simulink model "IEEE9Buses"  (R2024b)
settings: Solver=FixedStepAuto  StartTime=0  StopTime=5  FixedStep=1e-6  RelTol=1e-3
values from neighbouring files (symbols this model uses):
  SG_D_1_D = 0.01056    [SG9_parameters.m]
  SG_D_1_EnableSaturation = 0    [SG9_parameters.m]
  SG_D_1_f0 = 60    [SG9_parameters.m]
  SG_D_1_H = 7.5    [SG9_parameters.m]
  SG_D_1_K_A = 20    [SG9_parameters.m]
  SG_D_1_K_E = 1.000000e+1    (= 10)    [SG9_parameters.m]
  SG_D_1_K_F = 2.363    [SG9_parameters.m]
  SG_D_1_K_s = 5    [SG9_parameters.m]
  SG_D_1_R_a = 0.001088    [SG9_parameters.m]
  SG_D_1_S_A = 1    [SG9_parameters.m]
  SG_D_1_S_B = 0.103    [SG9_parameters.m]
  SG_D_1_S_N = 10.659857    [SG9_parameters.m]
  SG_D_1_SpeedPara = 200    [SG9_parameters.m]
  SG_D_1_T_0 = 0.720173    [SG9_parameters.m]
  SG_D_1_T_1 = 0.3    [SG9_parameters.m]
  SG_D_1_T_2 = 0.05    [SG9_parameters.m]
  SG_D_1_T_3 = 0.02    [SG9_parameters.m]
  SG_D_1_T_4 = 0.005    [SG9_parameters.m]
  SG_D_1_T_A = 0.02    [SG9_parameters.m]
  SG_D_1_T_dd = 8.000000e+0    (= 8)    [SG9_parameters.m]
  SG_D_1_T_ddd = 0.04    [SG9_parameters.m]
  SG_D_1_T_E = 0.314    [SG9_parameters.m]
  SG_D_1_T_F = 0.35    [SG9_parameters.m]
  SG_D_1_T_qd = 0.8    [SG9_parameters.m]
  SG_D_1_T_qdd = 0.02    [SG9_parameters.m]
  SG_D_1_T_speed = 0.1    [SG9_parameters.m]
  SG_D_1_T_w = 0.5    [SG9_parameters.m]
  SG_D_1_V_ref = 1.990276    [SG9_parameters.m]
  SG_D_1_w_ref = 376.991118    [SG9_parameters.m]
  SG_D_1_x_d = 1.9    [SG9_parameters.m]
  SG_D_1_x_dd = 0.302    [SG9_parameters.m]
  SG_D_1_x_ddd = 0.204    [SG9_parameters.m]
  SG_D_1_x_l = 0.05    [SG9_parameters.m]
  SG_D_1_x_q = 1.3    [SG9_parameters.m]
  SG_D_1_x_qd = 0.5    [SG9_parameters.m]
  SG_D_1_x_qdd = 0.3    [SG9_parameters.m]
  SG_D_2_D = 0.01056    [SG9_parameters.m]
  SG_D_2_EnableSaturation = 0    [SG9_parameters.m]
  SG_D_2_f0 = 60    [SG9_parameters.m]
  SG_D_2_H = 7.5    [SG9_parameters.m]
  SG_D_2_K_A = 20    [SG9_parameters.m]
  SG_D_2_K_E = 1.000000e+1    (= 10)    [SG9_parameters.m]
  SG_D_2_K_F = 2.363    [SG9_parameters.m]
  SG_D_2_K_s = 0.5    [SG9_parameters.m]
  SG_D_2_R_a = 0.001088    [SG9_parameters.m]
  SG_D_2_S_A = 1    [SG9_parameters.m]
  SG_D_2_S_B = 0.103    [SG9_parameters.m]
  SG_D_2_S_N = 10.659857    [SG9_parameters.m]
  SG_D_2_SpeedPara = 200    [SG9_parameters.m]
  SG_D_2_T_0 = 1.632913    [SG9_parameters.m]
  SG_D_2_T_1 = 0.2    [SG9_parameters.m]
  SG_D_2_T_2 = 0.05    [SG9_parameters.m]
  SG_D_2_T_3 = 0.02    [SG9_parameters.m]
  SG_D_2_T_4 = 0.005    [SG9_parameters.m]
  SG_D_2_T_A = 0.02    [SG9_parameters.m]
  SG_D_2_T_dd = 8.000000e+0    (= 8)    [SG9_parameters.m]
  SG_D_2_T_ddd = 0.04    [SG9_parameters.m]
  SG_D_2_T_E = 0.314    [SG9_parameters.m]
  SG_D_2_T_F = 0.35    [SG9_parameters.m]
  SG_D_2_T_qd = 0.8    [SG9_parameters.m]
  SG_D_2_T_qdd = 0.02    [SG9_parameters.m]
  SG_D_2_T_speed = 0.1    [SG9_parameters.m]
  SG_D_2_T_w = 0.5    [SG9_parameters.m]
  SG_D_2_V_ref = 2.662631    [SG9_parameters.m]
  SG_D_2_w_ref = 376.991118    [SG9_parameters.m]
  SG_D_2_x_d = 1.9    [SG9_parameters.m]
  SG_D_2_x_dd = 0.302    [SG9_parameters.m]
  SG_D_2_x_ddd = 0.204    [SG9_parameters.m]
  SG_D_2_x_l = 0.05    [SG9_parameters.m]
  SG_D_2_x_q = 1.3    [SG9_parameters.m]
  SG_D_2_x_qd = 0.5    [SG9_parameters.m]
  SG_D_2_x_qdd = 0.3    [SG9_parameters.m]
  SG_D_3_D = 0.01056    [SG9_parameters.m]
  SG_D_3_EnableSaturation = 0    [SG9_parameters.m]
  SG_D_3_f0 = 60    [SG9_parameters.m]
  SG_D_3_H = 7.5    [SG9_parameters.m]
  SG_D_3_K_A = 20    [SG9_parameters.m]
  SG_D_3_K_E = 1.000000e+1    (= 10)    [SG9_parameters.m]
  SG_D_3_K_F = 2.363    [SG9_parameters.m]
  SG_D_3_K_s = 0.5    [SG9_parameters.m]
  SG_D_3_R_a = 0.001088    [SG9_parameters.m]
  SG_D_3_S_A = 1    [SG9_parameters.m]
  SG_D_3_S_B = 0.103    [SG9_parameters.m]
  SG_D_3_S_N = 10.659857    [SG9_parameters.m]
  SG_D_3_SpeedPara = 200    [SG9_parameters.m]
  SG_D_3_T_0 = 0.850788    [SG9_parameters.m]
  SG_D_3_T_1 = 0.2    [SG9_parameters.m]
  SG_D_3_T_2 = 0.05    [SG9_parameters.m]
  SG_D_3_T_3 = 0.02    [SG9_parameters.m]
  SG_D_3_T_4 = 0.005    [SG9_parameters.m]
  SG_D_3_T_A = 0.02    [SG9_parameters.m]
  SG_D_3_T_dd = 8.000000e+0    (= 8)    [SG9_parameters.m]
  SG_D_3_T_ddd = 0.04    [SG9_parameters.m]
  SG_D_3_T_E = 0.314    [SG9_parameters.m]
  SG_D_3_T_F = 0.35    [SG9_parameters.m]
  SG_D_3_T_qd = 0.8    [SG9_parameters.m]
  SG_D_3_T_qdd = 0.02    [SG9_parameters.m]
  SG_D_3_T_speed = 0.1    [SG9_parameters.m]
  SG_D_3_T_w = 0.5    [SG9_parameters.m]
  SG_D_3_V_ref = 1.915682    [SG9_parameters.m]
  SG_D_3_w_ref = 376.991118    [SG9_parameters.m]
  SG_D_3_x_d = 1.9    [SG9_parameters.m]
  SG_D_3_x_dd = 0.302    [SG9_parameters.m]
  SG_D_3_x_ddd = 0.204    [SG9_parameters.m]
  SG_D_3_x_l = 0.05    [SG9_parameters.m]
  SG_D_3_x_q = 1.3    [SG9_parameters.m]
  SG_D_3_x_qd = 0.5    [SG9_parameters.m]
  SG_D_3_x_qdd = 0.3    [SG9_parameters.m]
(part 4 of 9)

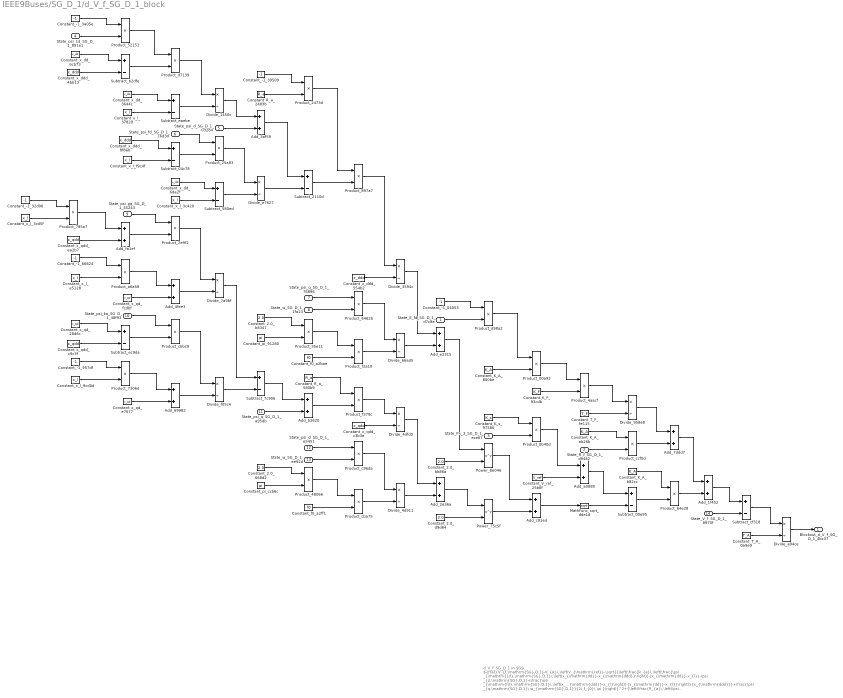
== system IEEE9Buses/SG_D_1/d_V_f_SG_D_1_block ==
  note: d_V_f_SG_D_1 in SG9
      | $-\frac{V_{f,\mathrm{SG},D,1}-K_{A}\,\left(V_{\mathrm{ref}}-\sqrt{{\left(\frac{R_{a}\,\left(\frac{\psi _{\mathrm{1d},\mathrm{SG},D,1}\,\left(x_{\mathrm{dd}}-x_{\mathrm{ddd}}\right)}{x_{\mathrm{dd}}-x_{l}}-\psi _{d,\mathrm{SG},D,1}+\frac{\psi _{\mathrm{fd},\mathrm{SG},D,1}\,\left(x_{\mathrm{ddd}}-x_{l}\right)}{x_{\mathrm{dd}}-x_{l}}\right)}{x_{\mathrm{ddd}}}+\frac{\psi _{q,\mathrm{SG},D,1}\,w_{\mathrm{SG},D,1}}{2\,f_{0}\,\pi }\right)}^2+{\left(\frac{R_{a}\,\left(\psi _{q,\mathrm{SG},D,1}+\frac{\psi _{\mathrm{gq},\mathrm{SG},D,1}\,\left(x_{l}-x_{\mathrm{qdd}}\right)}{x_{l}-x_{\mathrm{qd}}}+\frac{\psi _{\mathrm{kq},\mathrm{SG},D,1}\,\left(x_{\mathrm{qd}}-x_{\mathrm{qdd}}\right)}{x_{l}-x_{\mathrm{qd}}}\right)}{x_{\mathrm{qdd}}}+\frac{\psi _{d,\mathrm{SG},D,1}\,w_{\mathrm{SG},D,1}}{2\,f_{0}\,\pi }\right)}^2}+K_{s}\,\mathrm{Px}_{3,\mathrm{SG},D,1}\right)-K_{A}\,R_{f,\mathrm{SG},D,1}+\frac{E_{\mathrm{fd},\mathrm{SG},D,1}\,K_{A}\,K_{F}}{T_{F}}}{T_{A}}$
      | Automatically generated on 2025-09-12 21:31:27 .
  State_E_fd_SG_D_1_d7c8e : Inport
  State_R_f_SG_D_1_d9482 : Inport  Port=2
  State_Px_3_SG_D_1_ece67 : Inport  Port=3
  State_psi_1d_SG_D_1_891e1 : Inport  Port=4
  State_psi_d_SG_D_1_03284 : Inport  Port=5
  State_psi_fd_SG_D_1_16d3d : Inport  Port=6
  State_psi_q_SG_D_1_76896 : Inport  Port=7
  State_w_SG_D_1_1fa23 : Inport  Port=8
  State_psi_gq_SG_D_1_45243 : Inport  Port=9
  State_psi_kq_SG_D_1_48f93 : Inport  Port=10
  State_psi_q_SG_D_1_a95db : Inport  Port=11
  State_psi_d_SG_D_1_e5451 : Inport  Port=12
  State_w_SG_D_1_ee92d : Inport  Port=13
  State_V_f_SG_D_1_8970f : Inport  Port=14
  Add_1f452 : Sum
  Add_2e36a : Sum
  Add_3af59 : Sum
  Add_4fee3 : Sum
  Add_69982 : Sum
  Add_7ddd7 : Sum
  Add_a0880 : Sum
  Add_b2620 : Sum
  Add_c91ed : Sum
  Add_e2315 : Sum
  Add_fa1ef : Sum
  Constant_-1_04053 : Constant  Value=-1
  Constant_-1_32d06 : Constant  Value=-1
  Constant_-1_39509 : Constant  Value=-1
  Constant_-1_3a05e : Constant  Value=-1
  Constant_-1_66824 : Constant  Value=-1
  Constant_-1_957df : Constant  Value=-1
  Constant_2.0_668d2 : Constant  Value=2.0
  Constant_2.0_b8347 : Constant  Value=2.0
  Constant_2.0_bb86a : Constant  Value=2.0
  Constant_2.0_d9d64 : Constant  Value=2.0
  Constant_K_A_800be : Constant  Value=K_A
  Constant_K_A_ab26b : Constant  Value=K_A
  Constant_K_A_b82cc : Constant  Value=K_A
  Constant_K_F_93cdb : Constant  Value=K_F
  Constant_K_s_97580 : Constant  Value=K_s
  Constant_R_a_2483b : Constant  Value=R_a
  Constant_R_a_580b9 : Constant  Value=R_a
  Constant_T_A_0a9e9 : Constant  Value=T_A
  Constant_T_F_fe115 : Constant  Value=T_F
  Constant_V_ref_25b6f : Constant  Value=V_ref
  Constant_f0_a2bae : Constant  Value=f0
  Constant_f0_a2ff1 : Constant  Value=f0
  Constant_pi_91280 : Constant  Value=pi
  Constant_pi_ccb6c : Constant  Value=pi
  Constant_x_dd_3644c : Constant  Value=x_dd
  Constant_x_dd_6cb73 : Constant  Value=x_dd
  Constant_x_dd_6da2f : Constant  Value=x_dd
  Constant_x_ddd_4bb13 : Constant  Value=x_ddd
  Constant_x_ddd_554b2 : Constant  Value=x_ddd
  Constant_x_ddd_8f8ab : Constant  Value=x_ddd
  Constant_x_l_3782d : Constant  Value=x_l
  Constant_x_l_3c420 : Constant  Value=x_l
  Constant_x_l_3cd5f : Constant  Value=x_l
  Constant_x_l_9cd0d : Constant  Value=x_l
  Constant_x_l_e5128 : Constant  Value=x_l
  Constant_x_l_f9c4f : Constant  Value=x_l
  Constant_x_qd_28d6c : Constant  Value=x_qd
  Constant_x_qd_e7677 : Constant  Value=x_qd
  Constant_x_qd_fcdbf : Constant  Value=x_qd
  Constant_x_qdd_c3b3e : Constant  Value=x_qdd
  Constant_x_qdd_c9c3f : Constant  Value=x_qdd
  Constant_x_qdd_ea2b7 : Constant  Value=x_qdd
  Divide_1450c : Product  Inputs=*/
  Divide_3594c : Product  Inputs=*/
  Divide_4d911 : Product  Inputs=*/
  Divide_4dfd0 : Product  Inputs=*/
  Divide_66ad5 : Product  Inputs=*/
  Divide_7a9bf : Product  Inputs=*/
  Divide_958e8 : Product  Inputs=*/
  Divide_a94ce : Product  Inputs=*/
  Divide_e7627 : Product  Inputs=*/
  Divide_f05c4 : Product  Inputs=*/
  MathFunc_sqrt_dde1d : Sqrt
  Power_75c5f : Math  Operator=pow
  Power_8e046 : Math  Operator=pow
  Product_00a92 : Product
  Product_0b40d : Product
  Product_2473d : Product
  Product_25a83 : Product
  Product_2e9f2 : Product
  Product_35e11 : Product
  Product_48066 : Product
  Product_4aacf : Product
  Product_52151 : Product
  Product_6462b : Product
  Product_64e28 : Product
  Product_7306d : Product
  Product_785a7 : Product
  Product_897a7 : Product
  Product_a6a58 : Product
  Product_c96da : Product
  Product_cba75 : Product
  Product_cbbc9 : Product
  Product_ccf0d : Product
  Product_d7139 : Product
  Product_d98a2 : Product
  Product_f2a10 : Product
  Product_f379c : Product
  Subtract_00e95 : Sum  Inputs=+-
  Subtract_04c78 : Sum  Inputs=+-
  Subtract_2110d : Sum  Inputs=+-
  Subtract_580ed : Sum  Inputs=+-
  Subtract_7c906 : Sum  Inputs=+-
  Subtract_b2dfe : Sum  Inputs=+-
  Subtract_cf318 : Sum  Inputs=+-
  Subtract_eaebe : Sum  Inputs=+-
  Subtract_ec9da : Sum  Inputs=+-
  Blockout_d_V_f_SG_D_1_4bc37 : Outport
  wires:
  Constant_-1_957df/1 -> Product_7306d/1
  Constant_-1_32d06/1 -> Product_785a7/1
  State_psi_d_SG_D_1_e5451/1 -> Product_c96da/1
  Constant_x_qd_e7677/1 -> Add_69982/2
  Constant_x_qdd_ea2b7/1 -> Add_fa1ef/2
  State_w_SG_D_1_ee92d/1 -> Product_c96da/2
  Constant_x_l_3cd5f/1 -> Product_785a7/2
  Subtract_2110d/1 -> Product_897a7/2
  Constant_x_l_9cd0d/1 -> Product_7306d/2
  Constant_x_dd_6cb73/1 -> Subtract_b2dfe/1
  Constant_R_a_2483b/1 -> Product_2473d/2
  Constant_-1_3a05e/1 -> Product_52151/1
  Divide_e7627/1 -> Subtract_2110d/2
  Constant_x_ddd_4bb13/1 -> Subtract_b2dfe/2
  Add_69982/1 -> Divide_f05c4/2
  State_psi_1d_SG_D_1_891e1/1 -> Product_52151/2
  Add_4fee3/1 -> Divide_7a9bf/2
  Subtract_ec9da/1 -> Product_cbbc9/2
  Product_4aacf/1 -> Divide_958e8/1
  Product_35e11/1 -> Product_f2a10/1
  Product_785a7/1 -> Add_fa1ef/1
  Constant_-1_66824/1 -> Product_a6a58/1
  Constant_x_l_e5128/1 -> Product_a6a58/2
  Add_3af59/1 -> Subtract_2110d/1
  Constant_2.0_668d2/1 -> Product_48066/1
  Constant_x_qd_28d6c/1 -> Subtract_ec9da/1
  Product_52151/1 -> Product_d7139/1
  Constant_pi_ccb6c/1 -> Product_48066/2
  Constant_x_qdd_c9c3f/1 -> Subtract_ec9da/2
  Subtract_b2dfe/1 -> Product_d7139/2
  State_psi_q_SG_D_1_a95db/1 -> Add_b2620/2
  Constant_x_dd_3644c/1 -> Subtract_eaebe/1
  Constant_x_l_3782d/1 -> Subtract_eaebe/2
  Constant_x_ddd_8f8ab/1 -> Subtract_04c78/1
  Constant_x_l_f9c4f/1 -> Subtract_04c78/2
  State_psi_gq_SG_D_1_45243/1 -> Product_2e9f2/1
  Add_fa1ef/1 -> Product_2e9f2/2
  Product_a6a58/1 -> Add_4fee3/1
  Constant_x_qd_fcdbf/1 -> Add_4fee3/2
  Divide_1450c/1 -> Add_3af59/1
  Subtract_eaebe/1 -> Divide_1450c/2
  State_psi_kq_SG_D_1_48f93/1 -> Product_cbbc9/1
  Divide_a94ce/1 -> Blockout_d_V_f_SG_D_1_4bc37/1
  Product_7306d/1 -> Add_69982/1
  Product_d7139/1 -> Divide_1450c/1
  State_psi_fd_SG_D_1_16d3d/1 -> Product_25a83/1
  State_w_SG_D_1_1fa23/1 -> Product_6462b/2
  Subtract_04c78/1 -> Product_25a83/2
  Constant_x_dd_6da2f/1 -> Subtract_580ed/1
  Constant_x_l_3c420/1 -> Subtract_580ed/2
  Product_2e9f2/1 -> Divide_7a9bf/1
  Product_2473d/1 -> Product_897a7/1
  Product_cbbc9/1 -> Divide_f05c4/1
  State_psi_d_SG_D_1_03284/1 -> Add_3af59/2
  Product_25a83/1 -> Divide_e7627/1
  Subtract_580ed/1 -> Divide_e7627/2
  Divide_7a9bf/1 -> Subtract_7c906/1
  Divide_f05c4/1 -> Subtract_7c906/2
  Constant_-1_39509/1 -> Product_2473d/1
  Constant_2.0_b8347/1 -> Product_35e11/1
  Constant_pi_91280/1 -> Product_35e11/2
  Subtract_7c906/1 -> Add_b2620/1
  State_psi_q_SG_D_1_76896/1 -> Product_6462b/1
  Constant_f0_a2bae/1 -> Product_f2a10/2
  Constant_R_a_580b9/1 -> Product_f379c/1
  Add_b2620/1 -> Product_f379c/2
  Product_48066/1 -> Product_cba75/1
  Power_8e046/1 -> Add_c91ed/1
  Constant_f0_a2ff1/1 -> Product_cba75/2
  Product_897a7/1 -> Divide_3594c/1
  Constant_x_ddd_554b2/1 -> Divide_3594c/2
  Product_6462b/1 -> Divide_66ad5/1
  Product_f2a10/1 -> Divide_66ad5/2
  Product_f379c/1 -> Divide_4dfd0/1
  Constant_x_qdd_c3b3e/1 -> Divide_4dfd0/2
  Product_c96da/1 -> Divide_4d911/1
  Product_cba75/1 -> Divide_4d911/2
  Divide_3594c/1 -> Add_e2315/1
  Divide_66ad5/1 -> Add_e2315/2
  Divide_4dfd0/1 -> Add_2e36a/1
  Divide_4d911/1 -> Add_2e36a/2
  Constant_-1_04053/1 -> Product_d98a2/1
  State_E_fd_SG_D_1_d7c8e/1 -> Product_d98a2/2
  Add_e2315/1 -> Power_8e046/1
  Constant_2.0_bb86a/1 -> Power_8e046/2
  Add_2e36a/1 -> Power_75c5f/1
  Constant_2.0_d9d64/1 -> Power_75c5f/2
  Product_d98a2/1 -> Product_00a92/1
  Constant_K_A_800be/1 -> Product_00a92/2
  Constant_K_s_97580/1 -> Product_0b40d/1
  State_Px_3_SG_D_1_ece67/1 -> Product_0b40d/2
  Power_75c5f/1 -> Add_c91ed/2
  Divide_958e8/1 -> Add_7ddd7/1
  Product_00a92/1 -> Product_4aacf/1
  Constant_K_F_93cdb/1 -> Product_4aacf/2
  Product_0b40d/1 -> Add_a0880/1
  Constant_V_ref_25b6f/1 -> Add_a0880/2
  Add_c91ed/1 -> MathFunc_sqrt_dde1d/1
  Constant_T_F_fe115/1 -> Divide_958e8/2
  Constant_K_A_ab26b/1 -> Product_ccf0d/1
  State_R_f_SG_D_1_d9482/1 -> Product_ccf0d/2
  Add_a0880/1 -> Subtract_00e95/1
  MathFunc_sqrt_dde1d/1 -> Subtract_00e95/2
  Constant_T_A_0a9e9/1 -> Divide_a94ce/2
  Product_ccf0d/1 -> Add_7ddd7/2
  Constant_K_A_b82cc/1 -> Product_64e28/1
  Subtract_00e95/1 -> Product_64e28/2
  Add_7ddd7/1 -> Add_1f452/1
  Product_64e28/1 -> Add_1f452/2
  Add_1f452/1 -> Subtract_cf318/1
  State_V_f_SG_D_1_8970f/1 -> Subtract_cf318/2
  Subtract_cf318/1 -> Divide_a94ce/1

== system IEEE9Buses/SG_D_1/d_psi_1d_SG_D_1_block ==
  note: d_psi_1d_SG_D_1 in SG9
      | $-\frac{\psi _{\mathrm{1d},\mathrm{SG},D,1}-\psi _{\mathrm{fd},\mathrm{SG},D,1}+\frac{\left(x_{\mathrm{dd}}-x_{l}\right)\,\left(\frac{\psi _{\mathrm{1d},\mathrm{SG},D,1}\,\left(x_{\mathrm{dd}}-x_{\mathrm{ddd}}\right)}{x_{\mathrm{dd}}-x_{l}}-\psi _{d,\mathrm{SG},D,1}+\frac{\psi _{\mathrm{fd},\mathrm{SG},D,1}\,\left(x_{\mathrm{ddd}}-x_{l}\right)}{x_{\mathrm{dd}}-x_{l}}\right)}{x_{\mathrm{ddd}}}}{T_{\mathrm{ddd}}}$
      | Automatically generated on 2025-09-12 21:31:05 .
  State_psi_1d_SG_D_1_d2762 : Inport
  State_psi_fd_SG_D_1_bca21 : Inport  Port=2
  State_psi_1d_SG_D_1_c520a : Inport  Port=3
  State_psi_d_SG_D_1_3f3ac : Inport  Port=4
  State_psi_fd_SG_D_1_eccee : Inport  Port=5
  Add_b1279 : Sum
  Add_c201e : Sum
  Add_cfc23 : Sum
  Constant_-1_296e1 : Constant  Value=-1
  Constant_-1_5c271 : Constant  Value=-1
  Constant_T_ddd_caaec : Constant  Value=T_ddd
  Constant_x_dd_2b56b : Constant  Value=x_dd
  Constant_x_dd_87b87 : Constant  Value=x_dd
  Constant_x_dd_8f6dc : Constant  Value=x_dd
  Constant_x_dd_c90dd : Constant  Value=x_dd
  Constant_x_ddd_16ccc : Constant  Value=x_ddd
  Constant_x_ddd_bf0c4 : Constant  Value=x_ddd
  Constant_x_ddd_d1635 : Constant  Value=x_ddd
  Constant_x_l_09e53 : Constant  Value=x_l
  Constant_x_l_48004 : Constant  Value=x_l
  Constant_x_l_58458 : Constant  Value=x_l
  Constant_x_l_bfbd3 : Constant  Value=x_l
  Divide_2506c : Product  Inputs=*/
  Divide_70d34 : Product  Inputs=*/
  Divide_77283 : Product  Inputs=*/
  Divide_cc347 : Product  Inputs=*/
  Product_15131 : Product
  Product_1d398 : Product
  Product_2cf84 : Product
  Product_4a14f : Product
  Product_e7278 : Product
  Subtract_15a9f : Sum  Inputs=+-
  Subtract_1ef53 : Sum  Inputs=+-
  Subtract_30208 : Sum  Inputs=+-
  Subtract_aaa5c : Sum  Inputs=+-
  Subtract_b8043 : Sum  Inputs=+-
  Subtract_efad1 : Sum  Inputs=+-
  Blockout_d_psi_1d_SG_D_1_4de60 : Outport
  wires:
  Product_15131/1 -> Product_4a14f/1
  Constant_-1_296e1/1 -> Product_15131/1
  Subtract_1ef53/1 -> Product_4a14f/2
  State_psi_1d_SG_D_1_c520a/1 -> Product_15131/2
  Subtract_b8043/1 -> Product_e7278/1
  State_psi_d_SG_D_1_3f3ac/1 -> Add_b1279/2
  Constant_x_dd_2b56b/1 -> Subtract_15a9f/1
  Constant_x_l_09e53/1 -> Subtract_b8043/2
  Constant_x_dd_8f6dc/1 -> Subtract_1ef53/1
  Subtract_30208/1 -> Product_2cf84/2
  Constant_x_l_48004/1 -> Subtract_15a9f/2
  Divide_2506c/1 -> Subtract_efad1/2
  Constant_x_ddd_16ccc/1 -> Subtract_1ef53/2
  Constant_x_ddd_bf0c4/1 -> Subtract_30208/1
  Constant_x_l_bfbd3/1 -> Subtract_30208/2
  Add_cfc23/1 -> Add_c201e/1
  Product_4a14f/1 -> Divide_77283/1
  Divide_cc347/1 -> Add_c201e/2
  Subtract_15a9f/1 -> Divide_77283/2
  State_psi_fd_SG_D_1_eccee/1 -> Product_2cf84/1
  Constant_x_dd_c90dd/1 -> Subtract_aaa5c/1
  Constant_x_l_58458/1 -> Subtract_aaa5c/2
  Constant_x_ddd_d1635/1 -> Divide_cc347/2
  Subtract_efad1/1 -> Product_e7278/2
  Divide_77283/1 -> Add_b1279/1
  Product_2cf84/1 -> Divide_2506c/1
  Subtract_aaa5c/1 -> Divide_2506c/2
  Product_e7278/1 -> Divide_cc347/1
  Constant_x_dd_87b87/1 -> Subtract_b8043/1
  Add_b1279/1 -> Subtract_efad1/1
  Constant_-1_5c271/1 -> Product_1d398/1
  State_psi_1d_SG_D_1_d2762/1 -> Product_1d398/2
  Product_1d398/1 -> Add_cfc23/1
  State_psi_fd_SG_D_1_bca21/1 -> Add_cfc23/2
  Add_c201e/1 -> Divide_70d34/1
  Constant_T_ddd_caaec/1 -> Divide_70d34/2
  Divide_70d34/1 -> Blockout_d_psi_1d_SG_D_1_4de60/1

== system IEEE9Buses/SG_D_1/d_psi_d_SG_D_1_block ==
  note: d_psi_d_SG_D_1 in SG9
      | $2\,\pi \,f_{0}\,\left(v_{d,\mathrm{SG},D,1}\,\sin\left(\theta _{\mathrm{SG},D,1}\right)-v_{q,\mathrm{SG},D,1}\,\cos\left(\theta _{\mathrm{SG},D,1}\right)+\frac{R_{a}\,\left(\frac{\psi _{\mathrm{1d},\mathrm{SG},D,1}\,\left(x_{\mathrm{dd}}-x_{\mathrm{ddd}}\right)}{x_{\mathrm{dd}}-x_{l}}-\psi _{d,\mathrm{SG},D,1}+\frac{\psi _{\mathrm{fd},\mathrm{SG},D,1}\,\left(x_{\mathrm{ddd}}-x_{l}\right)}{x_{\mathrm{dd}}-x_{l}}\right)}{x_{\mathrm{ddd}}}+\frac{\psi _{q,\mathrm{SG},D,1}\,w_{\mathrm{SG},D,1}}{2\,f_{0}\,\pi }\right)$
      | Automatically generated on 2025-09-12 21:30:56 .
  State_psi_1d_SG_D_1_86041 : Inport
  State_psi_d_SG_D_1_dbe44 : Inport  Port=2
  State_psi_fd_SG_D_1_6e896 : Inport  Port=3
  Input_v_d_SG_D_1_19f90 : Inport  Port=4
  State_theta_SG_D_1_15a2a : Inport  Port=5
  Input_v_q_SG_D_1_67e4a : Inport  Port=6
  State_theta_SG_D_1_2debe : Inport  Port=7
  State_psi_q_SG_D_1_4f741 : Inport  Port=8
  State_w_SG_D_1_13bdb : Inport  Port=9
  Add_51bf5 : Sum
  Add_5a4e2 : Sum
  Constant_-1_86b72 : Constant  Value=-1
  Constant_-2.0_180c6 : Constant  Value=-2.0
  Constant_2.0_e7900 : Constant  Value=2.0
  Constant_R_a_4c0ac : Constant  Value=R_a
  Constant_f0_3c565 : Constant  Value=f0
  Constant_f0_a234f : Constant  Value=f0
  Constant_pi_33d76 : Constant  Value=pi
  Constant_pi_5f677 : Constant  Value=pi
  Constant_x_dd_5ee26 : Constant  Value=x_dd
  Constant_x_dd_bfc30 : Constant  Value=x_dd
  Constant_x_dd_dc9dd : Constant  Value=x_dd
  Constant_x_ddd_43fba : Constant  Value=x_ddd
  Constant_x_ddd_75169 : Constant  Value=x_ddd
  Constant_x_ddd_d754c : Constant  Value=x_ddd
  Constant_x_l_4ff12 : Constant  Value=x_l
  Constant_x_l_79896 : Constant  Value=x_l
  Constant_x_l_82ac6 : Constant  Value=x_l
  Divide_5216b : Product  Inputs=*/
  Divide_5b670 : Product  Inputs=*/
  Divide_816d9 : Product  Inputs=*/
  Divide_f246b : Product  Inputs=*/
  MathFunc_cos_15b49 : Trigonometry  Operator=cos
  MathFunc_sin_0787e : Trigonometry
  Product_06b68 : Product
  Product_11279 : Product
  Product_27c5b : Product
  Product_28ed5 : Product
  Product_3b359 : Product
  Product_3ce3c : Product
  Product_44fc3 : Product
  Product_70878 : Product
  Product_7e125 : Product
  Product_d0240 : Product
  Product_d34c7 : Product
  Product_f3a48 : Product
  Subtract_0408f : Sum  Inputs=+-
  Subtract_0ef44 : Sum  Inputs=+-
  Subtract_112a7 : Sum  Inputs=+-
  Subtract_4ad5b : Sum  Inputs=+-
  Subtract_54635 : Sum  Inputs=+-
  Subtract_78ef5 : Sum  Inputs=+-
  Subtract_c5ec9 : Sum  Inputs=+-
  Blockout_d_psi_d_SG_D_1_534f2 : Outport
  wires:
  Add_51bf5/1 -> Subtract_0ef44/1
  Product_d34c7/1 -> Divide_5b670/1
  Subtract_c5ec9/1 -> Product_d34c7/2
  Divide_5b670/1 -> Add_51bf5/1
  Product_27c5b/1 -> Product_d34c7/1
  Constant_x_ddd_d754c/1 -> Subtract_c5ec9/2
  Constant_x_dd_dc9dd/1 -> Subtract_c5ec9/1
  State_psi_1d_SG_D_1_86041/1 -> Product_27c5b/2
  Constant_-1_86b72/1 -> Product_27c5b/1
  Product_f3a48/1 -> Divide_f246b/1
  Constant_x_l_4ff12/1 -> Subtract_4ad5b/2
  State_psi_d_SG_D_1_dbe44/1 -> Add_51bf5/2
  Constant_x_dd_bfc30/1 -> Subtract_4ad5b/1
  Constant_x_ddd_43fba/1 -> Subtract_78ef5/1
  Constant_x_l_82ac6/1 -> Subtract_78ef5/2
  Subtract_4ad5b/1 -> Divide_5b670/2
  State_psi_fd_SG_D_1_6e896/1 -> Product_f3a48/1
  Constant_x_ddd_75169/1 -> Divide_816d9/2
  Subtract_78ef5/1 -> Product_f3a48/2
  Product_7e125/1 -> Subtract_112a7/2
  Constant_x_dd_5ee26/1 -> Subtract_54635/1
  Constant_x_l_79896/1 -> Subtract_54635/2
  Subtract_54635/1 -> Divide_f246b/2
  Divide_f246b/1 -> Subtract_0ef44/2
  Constant_R_a_4c0ac/1 -> Product_d0240/1
  Subtract_0ef44/1 -> Product_d0240/2
  MathFunc_cos_15b49/1 -> Product_44fc3/2
  State_theta_SG_D_1_15a2a/1 -> MathFunc_sin_0787e/1
  Divide_816d9/1 -> Subtract_112a7/1
  Product_d0240/1 -> Divide_816d9/1
  MathFunc_sin_0787e/1 -> Product_7e125/2
  Input_v_d_SG_D_1_19f90/1 -> Product_7e125/1
  Product_06b68/1 -> Blockout_d_psi_d_SG_D_1_534f2/1
  Product_11279/1 -> Product_06b68/1
  Product_3ce3c/1 -> Product_11279/1
  State_theta_SG_D_1_2debe/1 -> MathFunc_cos_15b49/1
  Constant_2.0_e7900/1 -> Product_70878/1
  Constant_pi_33d76/1 -> Product_70878/2
  Input_v_q_SG_D_1_67e4a/1 -> Product_44fc3/1
  Constant_f0_a234f/1 -> Product_11279/2
  State_psi_q_SG_D_1_4f741/1 -> Product_28ed5/1
  State_w_SG_D_1_13bdb/1 -> Product_28ed5/2
  Product_70878/1 -> Product_3b359/1
  Constant_pi_5f677/1 -> Product_3ce3c/2
  Constant_f0_3c565/1 -> Product_3b359/2
  Constant_-2.0_180c6/1 -> Product_3ce3c/1
  Add_5a4e2/1 -> Subtract_0408f/1
  Subtract_112a7/1 -> Add_5a4e2/1
  Product_44fc3/1 -> Add_5a4e2/2
  Product_28ed5/1 -> Divide_5216b/1
  Product_3b359/1 -> Divide_5216b/2
  Divide_5216b/1 -> Subtract_0408f/2
  Subtract_0408f/1 -> Product_06b68/2

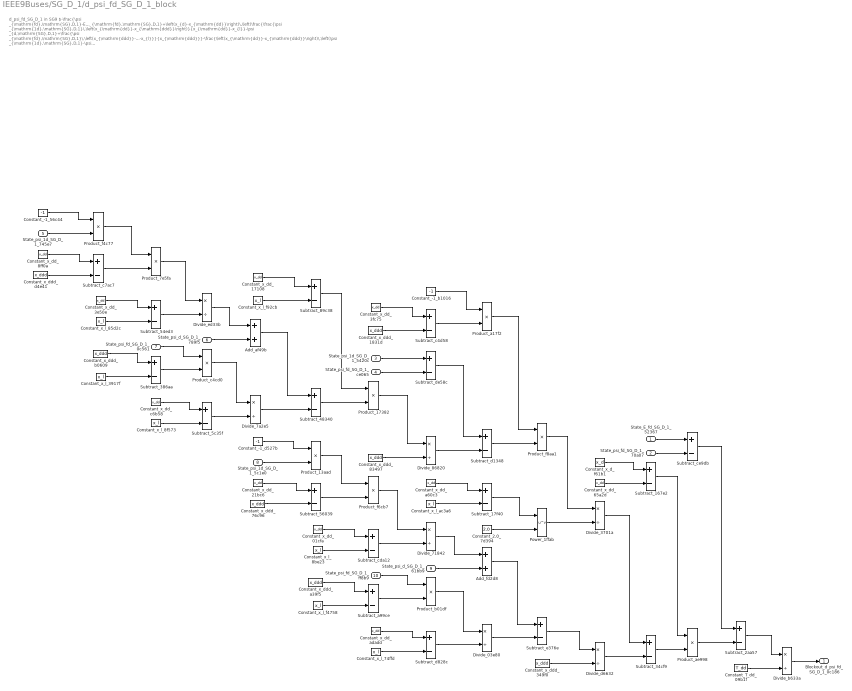
== system IEEE9Buses/SG_D_1/d_psi_fd_SG_D_1_block ==
  note: d_psi_fd_SG_D_1 in SG9
      | $-\frac{\psi _{\mathrm{fd},\mathrm{SG},D,1}-E_{\mathrm{fd},\mathrm{SG},D,1}+\left(x_{d}-x_{\mathrm{dd}}\right)\,\left(\frac{\frac{\psi _{\mathrm{1d},\mathrm{SG},D,1}\,\left(x_{\mathrm{dd}}-x_{\mathrm{ddd}}\right)}{x_{\mathrm{dd}}-x_{l}}-\psi _{d,\mathrm{SG},D,1}+\frac{\psi _{\mathrm{fd},\mathrm{SG},D,1}\,\left(x_{\mathrm{ddd}}-x_{l}\right)}{x_{\mathrm{dd}}-x_{l}}}{x_{\mathrm{ddd}}}-\frac{\left(x_{\mathrm{dd}}-x_{\mathrm{ddd}}\right)\,\left(\psi _{\mathrm{1d},\mathrm{SG},D,1}-\psi _{\mathrm{fd},\mathrm{SG},D,1}+\frac{\left(x_{\mathrm{dd}}-x_{l}\right)\,\left(\frac{\psi _{\mathrm{1d},\mathrm{SG},D,1}\,\left(x_{\mathrm{dd}}-x_{\mathrm{ddd}}\right)}{x_{\mathrm{dd}}-x_{l}}-\psi _{d,\mathrm{SG},D,1}+\frac{\psi _{\mathrm{fd},\mathrm{SG},D,1}\,\left(x_{\mathrm{ddd}}-x_{l}\right)}{x_{\mathrm{dd}}-x_{l}}\right)}{x_{\mathrm{ddd}}}\right)}{{\left(x_{\mathrm{dd}}-x_{l}\right)}^2}\right)}{T_{\mathrm{dd}}}$
      | Automatically generated on 2025-09-12 21:31:02 .
  State_E_fd_SG_D_1_52367 : Inport
  State_psi_fd_SG_D_1_70a07 : Inport  Port=2
  State_psi_1d_SG_D_1_5420c : Inport  Port=3
  State_psi_fd_SG_D_1_ce065 : Inport  Port=4
  State_psi_1d_SG_D_1_745e7 : Inport  Port=5
  State_psi_d_SG_D_1_789f5 : Inport  Port=6
  State_psi_fd_SG_D_1_0c561 : Inport  Port=7
  State_psi_1d_SG_D_1_5c1e0 : Inport  Port=8
  State_psi_d_SG_D_1_61bb9 : Inport  Port=9
  State_psi_fd_SG_D_1_ff8b9 : Inport  Port=10
  Add_af49b : Sum
  Add_fd2d8 : Sum
  Constant_-1_56c44 : Constant  Value=-1
  Constant_-1_b1016 : Constant  Value=-1
  Constant_-1_d527b : Constant  Value=-1
  Constant_2.0_7d394 : Constant  Value=2.0
  Constant_T_dd_09b1f : Constant  Value=T_dd
  Constant_x_d_f61b1 : Constant  Value=x_d
  Constant_x_dd_01cfa : Constant  Value=x_dd
  Constant_x_dd_17108 : Constant  Value=x_dd
  Constant_x_dd_21bc6 : Constant  Value=x_dd
  Constant_x_dd_3e50e : Constant  Value=x_dd
  Constant_x_dd_3fc75 : Constant  Value=x_dd
  Constant_x_dd_65a2d : Constant  Value=x_dd
  Constant_x_dd_8ff0a : Constant  Value=x_dd
  Constant_x_dd_a60c3 : Constant  Value=x_dd
  Constant_x_dd_adadd : Constant  Value=x_dd
  Constant_x_dd_c6b58 : Constant  Value=x_dd
  Constant_x_ddd_1831d : Constant  Value=x_ddd
  Constant_x_ddd_349f0 : Constant  Value=x_ddd
  Constant_x_ddd_76c96 : Constant  Value=x_ddd
  Constant_x_ddd_83497 : Constant  Value=x_ddd
  Constant_x_ddd_a39f5 : Constant  Value=x_ddd
  Constant_x_ddd_b0609 : Constant  Value=x_ddd
  Constant_x_ddd_d4e41 : Constant  Value=x_ddd
  Constant_x_l_3917f : Constant  Value=x_l
  Constant_x_l_74ffd : Constant  Value=x_l
  Constant_x_l_85d2c : Constant  Value=x_l
  Constant_x_l_8be23 : Constant  Value=x_l
  Constant_x_l_8f573 : Constant  Value=x_l
  Constant_x_l_ac3a6 : Constant  Value=x_l
  Constant_x_l_f4758 : Constant  Value=x_l
  Constant_x_l_f92cb : Constant  Value=x_l
  Divide_03e80 : Product  Inputs=*/
  Divide_3701a : Product  Inputs=*/
  Divide_71842 : Product  Inputs=*/
  Divide_7a2e5 : Product  Inputs=*/
  Divide_86820 : Product  Inputs=*/
  Divide_b633a : Product  Inputs=*/
  Divide_d6632 : Product  Inputs=*/
  Divide_ed33b : Product  Inputs=*/
  Power_1ffab : Math  Operator=pow
  Product_13aad : Product
  Product_17382 : Product
  Product_7e5fa : Product
  Product_a17f2 : Product
  Product_ae998 : Product
  Product_b01df : Product
  Product_c4cd0 : Product
  Product_f4c77 : Product
  Product_f6cb7 : Product
  Product_f8aa1 : Product
  Subtract_167e2 : Sum  Inputs=+-
  Subtract_17f40 : Sum  Inputs=+-
  Subtract_2aa57 : Sum  Inputs=+-
  Subtract_34cf9 : Sum  Inputs=+-
  Subtract_386aa : Sum  Inputs=+-
  Subtract_48340 : Sum  Inputs=+-
  Subtract_54ed3 : Sum  Inputs=+-
  Subtract_56039 : Sum  Inputs=+-
  Subtract_5c35f : Sum  Inputs=+-
  Subtract_89c38 : Sum  Inputs=+-
  Subtract_a99ce : Sum  Inputs=+-
  Subtract_c4d58 : Sum  Inputs=+-
  Subtract_c7ac7 : Sum  Inputs=+-
  Subtract_cda12 : Sum  Inputs=+-
  Subtract_ce9db : Sum  Inputs=+-
  Subtract_d1348 : Sum  Inputs=+-
  Subtract_d828c : Sum  Inputs=+-
  Subtract_de58c : Sum  Inputs=+-
  Subtract_e376e : Sum  Inputs=+-
  Blockout_d_psi_fd_SG_D_1_0c186 : Outport
  wires:
  State_psi_d_SG_D_1_789f5/1 -> Add_af49b/2
  Constant_x_dd_3e50e/1 -> Subtract_54ed3/1
  Product_7e5fa/1 -> Divide_ed33b/1
  Subtract_c7ac7/1 -> Product_7e5fa/2
  Subtract_48340/1 -> Product_17382/2
  Product_f4c77/1 -> Product_7e5fa/1
  Constant_x_dd_8ff0a/1 -> Subtract_c7ac7/1
  Constant_x_l_f92cb/1 -> Subtract_89c38/2
  Constant_-1_56c44/1 -> Product_f4c77/1
  Subtract_89c38/1 -> Product_17382/1
  Constant_x_l_85d2c/1 -> Subtract_54ed3/2
  Constant_x_ddd_d4e41/1 -> Subtract_c7ac7/2
  State_psi_1d_SG_D_1_745e7/1 -> Product_f4c77/2
  Constant_x_ddd_b0609/1 -> Subtract_386aa/1
  Constant_x_l_3917f/1 -> Subtract_386aa/2
  State_E_fd_SG_D_1_52367/1 -> Subtract_ce9db/1
  Divide_ed33b/1 -> Add_af49b/1
  Subtract_54ed3/1 -> Divide_ed33b/2
  State_psi_fd_SG_D_1_0c561/1 -> Product_c4cd0/1
  Constant_x_ddd_83497/1 -> Divide_86820/2
  Subtract_386aa/1 -> Product_c4cd0/2
  Constant_x_dd_c6b58/1 -> Subtract_5c35f/1
  Constant_x_dd_a60c3/1 -> Subtract_17f40/1
  State_psi_fd_SG_D_1_70a07/1 -> Subtract_ce9db/2
  Constant_x_l_8f573/1 -> Subtract_5c35f/2
  Product_c4cd0/1 -> Divide_7a2e5/1
  Constant_-1_b1016/1 -> Product_a17f2/1
  Subtract_5c35f/1 -> Divide_7a2e5/2
  Constant_x_dd_17108/1 -> Subtract_89c38/1
  Add_af49b/1 -> Subtract_48340/1
  Constant_x_l_ac3a6/1 -> Subtract_17f40/2
  Divide_7a2e5/1 -> Subtract_48340/2
  Divide_3701a/1 -> Subtract_34cf9/1
  Constant_-1_d527b/1 -> Product_13aad/1
  State_psi_1d_SG_D_1_5c1e0/1 -> Product_13aad/2
  Constant_x_dd_21bc6/1 -> Subtract_56039/1
  Subtract_c4d58/1 -> Product_a17f2/2
  Constant_x_ddd_76c96/1 -> Subtract_56039/2
  Product_13aad/1 -> Product_f6cb7/1
  Constant_2.0_7d394/1 -> Power_1ffab/2
  Product_f6cb7/1 -> Divide_71842/1
  Subtract_34cf9/1 -> Product_ae998/2
  Subtract_56039/1 -> Product_f6cb7/2
  State_psi_d_SG_D_1_61bb9/1 -> Add_fd2d8/2
  Constant_x_dd_01cfa/1 -> Subtract_cda12/1
  Constant_x_l_8be23/1 -> Subtract_cda12/2
  Constant_x_dd_3fc75/1 -> Subtract_c4d58/1
  Divide_86820/1 -> Subtract_d1348/2
  Constant_x_ddd_a39f5/1 -> Subtract_a99ce/1
  Constant_x_ddd_1831d/1 -> Subtract_c4d58/2
  Constant_x_l_f4758/1 -> Subtract_a99ce/2
  Subtract_a99ce/1 -> Product_b01df/2
  State_psi_1d_SG_D_1_5420c/1 -> Subtract_de58c/1
  Product_b01df/1 -> Divide_03e80/1
  State_psi_fd_SG_D_1_ce065/1 -> Subtract_de58c/2
  State_psi_fd_SG_D_1_ff8b9/1 -> Product_b01df/1
  Product_17382/1 -> Divide_86820/1
  Divide_71842/1 -> Add_fd2d8/1
  Subtract_cda12/1 -> Divide_71842/2
  Constant_x_dd_adadd/1 -> Subtract_d828c/1
  Constant_x_l_74ffd/1 -> Subtract_d828c/2
  Divide_03e80/1 -> Subtract_e376e/2
  Subtract_de58c/1 -> Subtract_d1348/1
  Subtract_d828c/1 -> Divide_03e80/2
  Subtract_d1348/1 -> Product_f8aa1/2
  Product_a17f2/1 -> Product_f8aa1/1
  Subtract_17f40/1 -> Power_1ffab/1
  Add_fd2d8/1 -> Subtract_e376e/1
  Product_f8aa1/1 -> Divide_3701a/1
  Power_1ffab/1 -> Divide_3701a/2
  Subtract_e376e/1 -> Divide_d6632/1
  Constant_x_ddd_349f0/1 -> Divide_d6632/2
  Constant_x_d_f61b1/1 -> Subtract_167e2/1
  Constant_x_dd_65a2d/1 -> Subtract_167e2/2
  Divide_d6632/1 -> Subtract_34cf9/2
  Subtract_167e2/1 -> Product_ae998/1
  Subtract_ce9db/1 -> Subtract_2aa57/1
  Product_ae998/1 -> Subtract_2aa57/2
  Subtract_2aa57/1 -> Divide_b633a/1
  Constant_T_dd_09b1f/1 -> Divide_b633a/2
  Divide_b633a/1 -> Blockout_d_psi_fd_SG_D_1_0c186/1

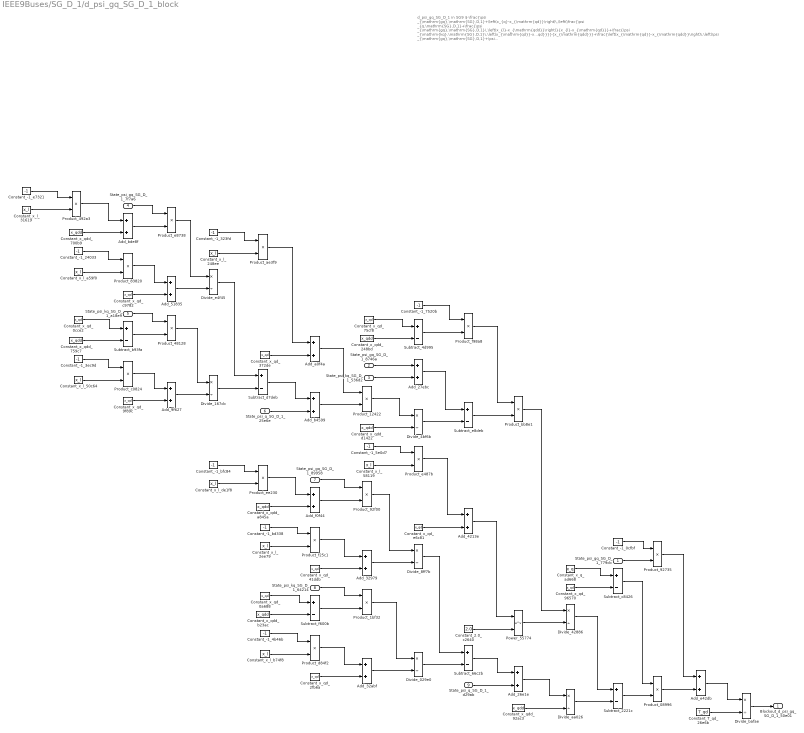
== system IEEE9Buses/SG_D_1/d_psi_gq_SG_D_1_block ==
  note: d_psi_gq_SG_D_1 in SG9
      | $-\frac{\psi _{\mathrm{gq},\mathrm{SG},D,1}+\left(x_{q}-x_{\mathrm{qd}}\right)\,\left(\frac{\psi _{q,\mathrm{SG},D,1}+\frac{\psi _{\mathrm{gq},\mathrm{SG},D,1}\,\left(x_{l}-x_{\mathrm{qdd}}\right)}{x_{l}-x_{\mathrm{qd}}}+\frac{\psi _{\mathrm{kq},\mathrm{SG},D,1}\,\left(x_{\mathrm{qd}}-x_{\mathrm{qdd}}\right)}{x_{l}-x_{\mathrm{qd}}}}{x_{\mathrm{qdd}}}+\frac{\left(x_{\mathrm{qd}}-x_{\mathrm{qdd}}\right)\,\left(\psi _{\mathrm{gq},\mathrm{SG},D,1}+\psi _{\mathrm{kq},\mathrm{SG},D,1}+\frac{\left(x_{l}-x_{\mathrm{qd}}\right)\,\left(\psi _{q,\mathrm{SG},D,1}+\frac{\psi _{\mathrm{gq},\mathrm{SG},D,1}\,\left(x_{l}-x_{\mathrm{qdd}}\right)}{x_{l}-x_{\mathrm{qd}}}+\frac{\psi _{\mathrm{kq},\mathrm{SG},D,1}\,\left(x_{\mathrm{qd}}-x_{\mathrm{qdd}}\right)}{x_{l}-x_{\mathrm{qd}}}\right)}{x_{\mathrm{qdd}}}\right)}{{\left(x_{l}-x_{\mathrm{qd}}\right)}^2}\right)}{T_{\mathrm{qd}}}$
      | Automatically generated on 2025-09-12 21:31:11 .
  State_psi_gq_SG_D_1_779cb : Inport
  State_psi_gq_SG_D_1_8746a : Inport  Port=2
  State_psi_kq_SG_D_1_536d2 : Inport  Port=3
  State_psi_gq_SG_D_1_7f7a6 : Inport  Port=4
  State_psi_kq_SG_D_1_a18e9 : Inport  Port=5
  State_psi_q_SG_D_1_25e6e : Inport  Port=6
  State_psi_gq_SG_D_1_89958 : Inport  Port=7
  State_psi_kq_SG_D_1_64214 : Inport  Port=8
  State_psi_q_SG_D_1_d29ab : Inport  Port=9
  Add_26e1e : Sum
  Add_27ebc : Sum
  Add_32979 : Sum
  Add_32abf : Sum
  Add_4213e : Sum
  Add_51835 : Sum
  Add_9f627 : Sum
  Add_a0f4a : Sum
  Add_b4599 : Sum
  Add_bde8f : Sum
  Add_e42db : Sum
  Add_f0f44 : Sum
  Constant_-1_0cfbf : Constant  Value=-1
  Constant_-1_24033 : Constant  Value=-1
  Constant_-1_323fd : Constant  Value=-1
  Constant_-1_3ec9d : Constant  Value=-1
  Constant_-1_4b46b : Constant  Value=-1
  Constant_-1_5e0d7 : Constant  Value=-1
  Constant_-1_7520b : Constant  Value=-1
  Constant_-1_bd338 : Constant  Value=-1
  Constant_-1_bfc84 : Constant  Value=-1
  Constant_-1_e7321 : Constant  Value=-1
  Constant_2.0_c2640 : Constant  Value=2.0
  Constant_T_qd_26e6b : Constant  Value=T_qd
  Constant_x_l_248ee : Constant  Value=x_l
  Constant_x_l_2ee79 : Constant  Value=x_l
  Constant_x_l_31619 : Constant  Value=x_l
  Constant_x_l_50c64 : Constant  Value=x_l
  Constant_x_l_58119 : Constant  Value=x_l
  Constant_x_l_a59f0 : Constant  Value=x_l
  Constant_x_l_b74f8 : Constant  Value=x_l
  Constant_x_l_de1f8 : Constant  Value=x_l
  Constant_x_q_ad668 : Constant  Value=x_q
  Constant_x_qd_0a688 : Constant  Value=x_qd
  Constant_x_qd_0cce2 : Constant  Value=x_qd
  Constant_x_qd_2fb6a : Constant  Value=x_qd
  Constant_x_qd_372de : Constant  Value=x_qd
  Constant_x_qd_41ddb : Constant  Value=x_qd
  Constant_x_qd_75cf8 : Constant  Value=x_qd
  Constant_x_qd_96570 : Constant  Value=x_qd
  Constant_x_qd_9f89c : Constant  Value=x_qd
  Constant_x_qd_c9782 : Constant  Value=x_qd
  Constant_x_qd_e6c81 : Constant  Value=x_qd
  Constant_x_qdd_248bd : Constant  Value=x_qdd
  Constant_x_qdd_700b9 : Constant  Value=x_qdd
  Constant_x_qdd_759c7 : Constant  Value=x_qdd
  Constant_x_qdd_92ac3 : Constant  Value=x_qdd
  Constant_x_qdd_a845a : Constant  Value=x_qdd
  Constant_x_qdd_b23ac : Constant  Value=x_qdd
  Constant_x_qdd_d1422 : Constant  Value=x_qdd
  Divide_029e0 : Product  Inputs=*/
  Divide_167cb : Product  Inputs=*/
  Divide_42886 : Product  Inputs=*/
  Divide_4bf6b : Product  Inputs=*/
  Divide_8ff7b : Product  Inputs=*/
  Divide_aa026 : Product  Inputs=*/
  Divide_bafae : Product  Inputs=*/
  Divide_e4f45 : Product  Inputs=*/
  Power_55774 : Math  Operator=pow
  Product_08996 : Product
  Product_{12422,48128,83820,92735} (4 alike) : Product
  Product_1bf32 : Product
  Product_492a3 : Product
  Product_92f00 : Product
  Product_ae3f9 : Product
  Product_bb8e1 : Product
  Product_c0824 : Product
  Product_d84f2 : Product
  Product_e487b : Product
  Product_e8738 : Product
  Product_ee230 : Product
  Product_f25c1 : Product
  Product_f98a8 : Product
  Subtract_2221c : Sum  Inputs=+-
  Subtract_4d995 : Sum  Inputs=+-
  Subtract_66c2b : Sum  Inputs=+-
  Subtract_b93fa : Sum  Inputs=+-
  Subtract_c8426 : Sum  Inputs=+-
  Subtract_d7deb : Sum  Inputs=+-
  Subtract_e8deb : Sum  Inputs=+-
  Subtract_f600b : Sum  Inputs=+-
  Blockout_d_psi_gq_SG_D_1_50e01 : Outport
  wires:
  State_psi_gq_SG_D_1_7f7a6/1 -> Product_e8738/1
  Constant_-1_24033/1 -> Product_83820/1
  Divide_e4f45/1 -> Subtract_d7deb/1
  Add_51835/1 -> Divide_e4f45/2
  Product_492a3/1 -> Add_bde8f/1
  Constant_x_qd_372de/1 -> Add_a0f4a/2
  Constant_-1_e7321/1 -> Product_492a3/1
  Constant_x_qdd_700b9/1 -> Add_bde8f/2
  Constant_x_l_a59f0/1 -> Product_83820/2
  Constant_x_l_31619/1 -> Product_492a3/2
  Constant_-1_3ec9d/1 -> Product_c0824/1
  Constant_x_qd_0cce2/1 -> Subtract_b93fa/1
  Constant_x_qdd_d1422/1 -> Divide_4bf6b/2
  Constant_x_l_50c64/1 -> Product_c0824/2
  Constant_x_qdd_759c7/1 -> Subtract_b93fa/2
  Subtract_d7deb/1 -> Add_b4599/1
  Add_bde8f/1 -> Product_e8738/2
  Product_e8738/1 -> Divide_e4f45/1
  Product_83820/1 -> Add_51835/1
  Constant_x_qd_c9782/1 -> Add_51835/2
  State_psi_kq_SG_D_1_a18e9/1 -> Product_48128/1
  Product_c0824/1 -> Add_9f627/1
  Subtract_b93fa/1 -> Product_48128/2
  Constant_x_qd_9f89c/1 -> Add_9f627/2
  Product_48128/1 -> Divide_167cb/1
  Add_9f627/1 -> Divide_167cb/2
  Constant_-1_7520b/1 -> Product_f98a8/1
  Constant_-1_323fd/1 -> Product_ae3f9/1
  Add_32979/1 -> Divide_8ff7b/2
  Product_d84f2/1 -> Add_32abf/1
  Subtract_f600b/1 -> Product_1bf32/2
  Constant_x_l_248ee/1 -> Product_ae3f9/2
  Divide_167cb/1 -> Subtract_d7deb/2
  Subtract_c8426/1 -> Product_08996/1
  Constant_-1_5e0d7/1 -> Product_e487b/1
  Constant_-1_bfc84/1 -> Product_ee230/1
  Constant_x_l_58119/1 -> Product_e487b/2
  Constant_x_l_de1f8/1 -> Product_ee230/2
  Constant_x_qd_41ddb/1 -> Add_32979/2
  Product_ae3f9/1 -> Add_a0f4a/1
  State_psi_q_SG_D_1_25e6e/1 -> Add_b4599/2
  Product_ee230/1 -> Add_f0f44/1
  Constant_x_qdd_a845a/1 -> Add_f0f44/2
  Constant_-1_bd338/1 -> Product_f25c1/1
  Constant_x_qd_2fb6a/1 -> Add_32abf/2
  Add_a0f4a/1 -> Product_12422/1
  Constant_x_l_2ee79/1 -> Product_f25c1/2
  Constant_-1_4b46b/1 -> Product_d84f2/1
  Constant_x_qd_0a688/1 -> Subtract_f600b/1
  Product_12422/1 -> Divide_4bf6b/1
  Constant_x_l_b74f8/1 -> Product_d84f2/2
  Divide_42886/1 -> Subtract_2221c/1
  Constant_x_qdd_b23ac/1 -> Subtract_f600b/2
  Add_b4599/1 -> Product_12422/2
  State_psi_gq_SG_D_1_89958/1 -> Product_92f00/1
  Add_f0f44/1 -> Product_92f00/2
  Product_f25c1/1 -> Add_32979/1
  State_psi_kq_SG_D_1_64214/1 -> Product_1bf32/1
  Add_32abf/1 -> Divide_029e0/2
  State_psi_gq_SG_D_1_8746a/1 -> Add_27ebc/1
  Constant_x_qd_75cf8/1 -> Subtract_4d995/1
  Constant_x_qdd_248bd/1 -> Subtract_4d995/2
  Product_1bf32/1 -> Divide_029e0/1
  State_psi_kq_SG_D_1_536d2/1 -> Add_27ebc/2
  Product_92f00/1 -> Divide_8ff7b/1
  Subtract_4d995/1 -> Product_f98a8/2
  Add_27ebc/1 -> Subtract_e8deb/1
  Divide_4bf6b/1 -> Subtract_e8deb/2
  Product_e487b/1 -> Add_4213e/1
  Constant_x_qd_e6c81/1 -> Add_4213e/2
  Divide_8ff7b/1 -> Subtract_66c2b/1
  Divide_029e0/1 -> Subtract_66c2b/2
  Product_f98a8/1 -> Product_bb8e1/1
  Subtract_e8deb/1 -> Product_bb8e1/2
  Add_4213e/1 -> Power_55774/1
  Constant_2.0_c2640/1 -> Power_55774/2
  Subtract_66c2b/1 -> Add_26e1e/1
  State_psi_q_SG_D_1_d29ab/1 -> Add_26e1e/2
  Product_bb8e1/1 -> Divide_42886/1
  Power_55774/1 -> Divide_42886/2
  Add_26e1e/1 -> Divide_aa026/1
  Constant_x_qdd_92ac3/1 -> Divide_aa026/2
  Constant_x_q_ad668/1 -> Subtract_c8426/1
  Constant_x_qd_96570/1 -> Subtract_c8426/2
  Divide_aa026/1 -> Subtract_2221c/2
  Constant_-1_0cfbf/1 -> Product_92735/1
  State_psi_gq_SG_D_1_779cb/1 -> Product_92735/2
  Subtract_2221c/1 -> Product_08996/2
  Product_92735/1 -> Add_e42db/1
  Product_08996/1 -> Add_e42db/2
  Add_e42db/1 -> Divide_bafae/1
  Constant_T_qd_26e6b/1 -> Divide_bafae/2
  Divide_bafae/1 -> Blockout_d_psi_gq_SG_D_1_50e01/1

== system IEEE9Buses/SG_D_1/d_psi_kq_SG_D_1_block ==
  note: d_psi_kq_SG_D_1 in SG9
      | $-\frac{\psi _{\mathrm{gq},\mathrm{SG},D,1}+\psi _{\mathrm{kq},\mathrm{SG},D,1}+\frac{\left(x_{l}-x_{\mathrm{qd}}\right)\,\left(\psi _{q,\mathrm{SG},D,1}+\frac{\psi _{\mathrm{gq},\mathrm{SG},D,1}\,\left(x_{l}-x_{\mathrm{qdd}}\right)}{x_{l}-x_{\mathrm{qd}}}+\frac{\psi _{\mathrm{kq},\mathrm{SG},D,1}\,\left(x_{\mathrm{qd}}-x_{\mathrm{qdd}}\right)}{x_{l}-x_{\mathrm{qd}}}\right)}{x_{\mathrm{qdd}}}}{T_{\mathrm{qdd}}}$
      | Automatically generated on 2025-09-12 21:31:13 .
  State_psi_gq_SG_D_1_14615 : Inport
  State_psi_kq_SG_D_1_2245f : Inport  Port=2
  State_psi_gq_SG_D_1_19905 : Inport  Port=3
  State_psi_kq_SG_D_1_6f435 : Inport  Port=4
  State_psi_q_SG_D_1_673e0 : Inport  Port=5
  Add_374a1 : Sum
  Add_43273 : Sum
  Add_76c08 : Sum
  Add_7ef94 : Sum
  Add_8a3b6 : Sum
  Add_8b2e8 : Sum
  Constant_-1_18001 : Constant  Value=-1
  Constant_-1_240b5 : Constant  Value=-1
  Constant_-1_8e20c : Constant  Value=-1
  Constant_-1_b9085 : Constant  Value=-1
  Constant_-1_d5deb : Constant  Value=-1
  Constant_T_qdd_a6e17 : Constant  Value=T_qdd
  Constant_x_l_1fed7 : Constant  Value=x_l
  Constant_x_l_26e27 : Constant  Value=x_l
  Constant_x_l_9a87b : Constant  Value=x_l
  Constant_x_l_efb03 : Constant  Value=x_l
  Constant_x_qd_14f23 : Constant  Value=x_qd
  Constant_x_qd_5a81c : Constant  Value=x_qd
  Constant_x_qd_5df5a : Constant  Value=x_qd
  Constant_x_qd_b981a : Constant  Value=x_qd
  Constant_x_qdd_c0805 : Constant  Value=x_qdd
  Constant_x_qdd_c4d4c : Constant  Value=x_qdd
  Constant_x_qdd_c4f7a : Constant  Value=x_qdd
  Divide_10e02 : Product  Inputs=*/
  Divide_7ad9d : Product  Inputs=*/
  Divide_b7563 : Product  Inputs=*/
  Divide_fd3ee : Product  Inputs=*/
  Product_3729c : Product
  Product_565b2 : Product
  Product_5877f : Product
  Product_6728a : Product
  Product_83c1b : Product
  Product_c0efa : Product
  Product_f4614 : Product
  Product_f57fc : Product
  Subtract_961c5 : Sum  Inputs=+-
  Subtract_97c9a : Sum  Inputs=+-
  Subtract_a5ff1 : Sum  Inputs=+-
  Blockout_d_psi_kq_SG_D_1_42599 : Outport
  wires:
  Product_3729c/1 -> Add_43273/1
  Constant_-1_b9085/1 -> Product_3729c/1
  Constant_x_l_9a87b/1 -> Product_3729c/2
  Constant_x_qdd_c0805/1 -> Add_43273/2
  Constant_-1_8e20c/1 -> Product_f4614/1
  Constant_x_qd_14f23/1 -> Subtract_a5ff1/1
  Constant_x_qd_5df5a/1 -> Add_8b2e8/2
  Constant_-1_240b5/1 -> Product_c0efa/1
  Constant_x_l_26e27/1 -> Product_f4614/2
  Constant_x_qdd_c4f7a/1 -> Subtract_a5ff1/2
  Constant_x_qd_b981a/1 -> Add_8a3b6/2
  Constant_x_l_1fed7/1 -> Product_c0efa/2
  Subtract_961c5/1 -> Add_76c08/1
  Product_565b2/1 -> Subtract_961c5/1
  State_psi_gq_SG_D_1_19905/1 -> Product_5877f/1
  Add_43273/1 -> Product_5877f/2
  Product_c0efa/1 -> Add_374a1/1
  Constant_x_qd_5a81c/1 -> Add_374a1/2
  State_psi_kq_SG_D_1_6f435/1 -> Product_83c1b/1
  Product_f4614/1 -> Add_8a3b6/1
  Subtract_a5ff1/1 -> Product_83c1b/2
  Product_5877f/1 -> Divide_b7563/1
  Add_374a1/1 -> Divide_b7563/2
  Product_83c1b/1 -> Divide_fd3ee/1
  Add_8a3b6/1 -> Divide_fd3ee/2
  Constant_-1_d5deb/1 -> Product_6728a/1
  Constant_x_l_efb03/1 -> Product_6728a/2
  Divide_b7563/1 -> Subtract_97c9a/1
  Divide_fd3ee/1 -> Subtract_97c9a/2
  Product_6728a/1 -> Add_8b2e8/1
  Add_7ef94/1 -> Product_f57fc/2
  Subtract_97c9a/1 -> Add_7ef94/1
  State_psi_q_SG_D_1_673e0/1 -> Add_7ef94/2
  Constant_-1_18001/1 -> Product_565b2/1
  State_psi_gq_SG_D_1_14615/1 -> Product_565b2/2
  Divide_10e02/1 -> Add_76c08/2
  Product_f57fc/1 -> Divide_10e02/1
  Add_8b2e8/1 -> Product_f57fc/1
  State_psi_kq_SG_D_1_2245f/1 -> Subtract_961c5/2
  Constant_x_qdd_c4d4c/1 -> Divide_10e02/2
  Add_76c08/1 -> Divide_7ad9d/1
  Constant_T_qdd_a6e17/1 -> Divide_7ad9d/2
  Divide_7ad9d/1 -> Blockout_d_psi_kq_SG_D_1_42599/1

== system IEEE9Buses/SG_D_1/d_psi_q_SG_D_1_block ==
  note: d_psi_q_SG_D_1 in SG9
      | $2\,\pi \,f_{0}\,\left(v_{d,\mathrm{SG},D,1}\,\cos\left(\theta _{\mathrm{SG},D,1}\right)+v_{q,\mathrm{SG},D,1}\,\sin\left(\theta _{\mathrm{SG},D,1}\right)-\frac{R_{a}\,\left(\psi _{q,\mathrm{SG},D,1}+\frac{\psi _{\mathrm{gq},\mathrm{SG},D,1}\,\left(x_{l}-x_{\mathrm{qdd}}\right)}{x_{l}-x_{\mathrm{qd}}}+\frac{\psi _{\mathrm{kq},\mathrm{SG},D,1}\,\left(x_{\mathrm{qd}}-x_{\mathrm{qdd}}\right)}{x_{l}-x_{\mathrm{qd}}}\right)}{x_{\mathrm{qdd}}}-\frac{\psi _{d,\mathrm{SG},D,1}\,w_{\mathrm{SG},D,1}}{2\,f_{0}\,\pi }\right)$
      | Automatically generated on 2025-09-12 21:30:59 .
  State_psi_gq_SG_D_1_d2ce1 : Inport
  State_psi_kq_SG_D_1_3d8c9 : Inport  Port=2
  State_psi_q_SG_D_1_a72f0 : Inport  Port=3
  Input_v_d_SG_D_1_612c6 : Inport  Port=4
  State_theta_SG_D_1_ab583 : Inport  Port=5
  Input_v_q_SG_D_1_0e1bb : Inport  Port=6
  State_theta_SG_D_1_4ed40 : Inport  Port=7
  State_psi_d_SG_D_1_23bff : Inport  Port=8
  State_w_SG_D_1_4a22e : Inport  Port=9
  Add_01763 : Sum
  Add_1d924 : Sum
  Add_64485 : Sum
  Add_6ab10 : Sum
  Add_bba13 : Sum
  Constant_-1_22a85 : Constant  Value=-1
  Constant_-1_2473f : Constant  Value=-1
  Constant_-1_63fca : Constant  Value=-1
  Constant_-2.0_20a91 : Constant  Value=-2.0
  Constant_2.0_d3b19 : Constant  Value=2.0
  Constant_R_a_7ee16 : Constant  Value=R_a
  Constant_f0_01622 : Constant  Value=f0
  Constant_f0_f1778 : Constant  Value=f0
  Constant_pi_5ca06 : Constant  Value=pi
  Constant_pi_a97e5 : Constant  Value=pi
  Constant_x_l_09fb3 : Constant  Value=x_l
  Constant_x_l_c30d5 : Constant  Value=x_l
  Constant_x_l_c4da3 : Constant  Value=x_l
  Constant_x_qd_2a05e : Constant  Value=x_qd
  Constant_x_qd_3097b : Constant  Value=x_qd
  Constant_x_qd_b7754 : Constant  Value=x_qd
  Constant_x_qdd_34540 : Constant  Value=x_qdd
  Constant_x_qdd_9cef3 : Constant  Value=x_qdd
  Constant_x_qdd_c624f : Constant  Value=x_qdd
  Divide_865e6 : Product  Inputs=*/
  Divide_8c45e : Product  Inputs=*/
  Divide_b872f : Product  Inputs=*/
  Divide_ec286 : Product  Inputs=*/
  MathFunc_cos_35a0f : Trigonometry  Operator=cos
  MathFunc_sin_16169 : Trigonometry
  Product_14d82 : Product
  Product_1de53 : Product
  Product_4663a : Product
  Product_49387 : Product
  Product_4952f : Product
  Product_61841 : Product
  Product_7592d : Product
  Product_7867b : Product
  Product_807c0 : Product
  Product_a3d27 : Product
  Product_b0b5f : Product
  Product_c0800 : Product
  Product_f52b7 : Product
  Product_fec05 : Product
  Subtract_3474a : Sum  Inputs=+-
  Subtract_38fff : Sum  Inputs=+-
  Subtract_40c74 : Sum  Inputs=+-
  Subtract_b26e4 : Sum  Inputs=+-
  Blockout_d_psi_q_SG_D_1_96a28 : Outport
  wires:
  Divide_865e6/1 -> Subtract_3474a/1
  Product_49387/1 -> Add_64485/1
  Constant_x_l_c4da3/1 -> Product_49387/2
  Constant_-1_22a85/1 -> Product_49387/1
  Constant_x_qdd_9cef3/1 -> Add_64485/2
  Constant_x_l_09fb3/1 -> Product_a3d27/2
  Constant_-1_2473f/1 -> Product_a3d27/1
  Constant_x_l_c30d5/1 -> Product_c0800/2
  Constant_x_qdd_34540/1 -> Subtract_b26e4/2
  State_psi_kq_SG_D_1_3d8c9/1 -> Product_f52b7/1
  Constant_-1_63fca/1 -> Product_c0800/1
  Constant_x_qd_2a05e/1 -> Subtract_b26e4/1
  State_psi_gq_SG_D_1_d2ce1/1 -> Product_807c0/1
  Product_7867b/1 -> Blockout_d_psi_q_SG_D_1_96a28/1
  Subtract_3474a/1 -> Add_1d924/1
  Product_807c0/1 -> Divide_865e6/1
  Add_64485/1 -> Product_807c0/2
  Divide_8c45e/1 -> Subtract_3474a/2
  Product_a3d27/1 -> Add_6ab10/1
  Constant_x_qd_b7754/1 -> Add_6ab10/2
  Constant_-2.0_20a91/1 -> Product_fec05/1
  Product_f52b7/1 -> Divide_8c45e/1
  Product_c0800/1 -> Add_01763/1
  Subtract_b26e4/1 -> Product_f52b7/2
  Constant_x_qd_3097b/1 -> Add_01763/2
  Add_6ab10/1 -> Divide_865e6/2
  Add_01763/1 -> Divide_8c45e/2
  Constant_f0_01622/1 -> Product_4663a/2
  State_psi_q_SG_D_1_a72f0/1 -> Add_1d924/2
  Product_61841/1 -> Product_1de53/1
  Constant_R_a_7ee16/1 -> Product_b0b5f/1
  Product_1de53/1 -> Divide_ec286/2
  Product_b0b5f/1 -> Divide_b872f/1
  Add_1d924/1 -> Product_b0b5f/2
  State_theta_SG_D_1_ab583/1 -> MathFunc_cos_35a0f/1
  Input_v_d_SG_D_1_612c6/1 -> Product_14d82/1
  Constant_x_qdd_c624f/1 -> Divide_b872f/2
  MathFunc_cos_35a0f/1 -> Product_14d82/2
  State_theta_SG_D_1_4ed40/1 -> MathFunc_sin_16169/1
  Divide_b872f/1 -> Subtract_38fff/1
  Constant_2.0_d3b19/1 -> Product_61841/1
  State_w_SG_D_1_4a22e/1 -> Product_7592d/2
  Constant_pi_a97e5/1 -> Product_61841/2
  Subtract_40c74/1 -> Add_bba13/1
  Product_14d82/1 -> Subtract_38fff/2
  Divide_ec286/1 -> Add_bba13/2
  Input_v_q_SG_D_1_0e1bb/1 -> Product_4952f/1
  MathFunc_sin_16169/1 -> Product_4952f/2
  Product_4952f/1 -> Subtract_40c74/2
  State_psi_d_SG_D_1_23bff/1 -> Product_7592d/1
  Constant_f0_f1778/1 -> Product_1de53/2
  Constant_pi_5ca06/1 -> Product_fec05/2
  Subtract_38fff/1 -> Subtract_40c74/1
  Product_7592d/1 -> Divide_ec286/1
  Product_fec05/1 -> Product_4663a/1
  Product_4663a/1 -> Product_7867b/1
  Add_bba13/1 -> Product_7867b/2

== system IEEE9Buses/SG_D_1/d_theta_SG_D_1_block ==
  note: d_theta_SG_D_1 in SG9
      | $w_{\mathrm{SG},D,1}-2\,\pi \,f_{0}$
      | Automatically generated on 2025-09-12 21:31:19 .
  State_w_SG_D_1_e3939 : Inport
  Add_ca348 : Sum
  Constant_-2.0_947f0 : Constant  Value=-2.0
  Constant_f0_6c0cd : Constant  Value=f0
  Constant_pi_d3054 : Constant  Value=pi
  Product_54d24 : Product
  Product_fe06d : Product
  Blockout_d_theta_SG_D_1_2b5f4 : Outport
  wires:
  State_w_SG_D_1_e3939/1 -> Add_ca348/2
  Constant_-2.0_947f0/1 -> Product_fe06d/1
  Constant_f0_6c0cd/1 -> Product_54d24/2
  Constant_pi_d3054/1 -> Product_fe06d/2
  Product_54d24/1 -> Add_ca348/1
  Product_fe06d/1 -> Product_54d24/1
  Add_ca348/1 -> Blockout_d_theta_SG_D_1_2b5f4/1
